simulink model "PolePlacement_Complete"  (R2021a)
settings: Solver=VariableStepAuto  StartTime=0.0  StopTime=10.0  RelTol=1e-3
values from neighbouring files (symbols this model uses):
  k = place(sysestc.A, sysestc.B, new_pole)    [PolePlacement.m]    (also in PolePlacement_Controller_script.m = place(A, B, new_pole); ppObs.m)
  Kr = 1/Kdc(1)    [PolePlacement.m]    (also in PolePlacement_Controller_script.m; ppObs.m)
  L = place(sysestc.A',sysestc.C', 10*new_pole)'    [PolePlacement.m]    (also in PolePlacement_Controller_script.m; ppObs.m)
  sysestc = d2c(sysest)    [PolePlacement.m]    (also in PolePlacement_Controller_script.m; ppObs.m)
undefined symbols (not defined in the file or in its folder): Kp, sigbuilder_block, Ti
libraries: cstblocks x1
settings Model: Creator=jesuc  LastModifiedBy=andre

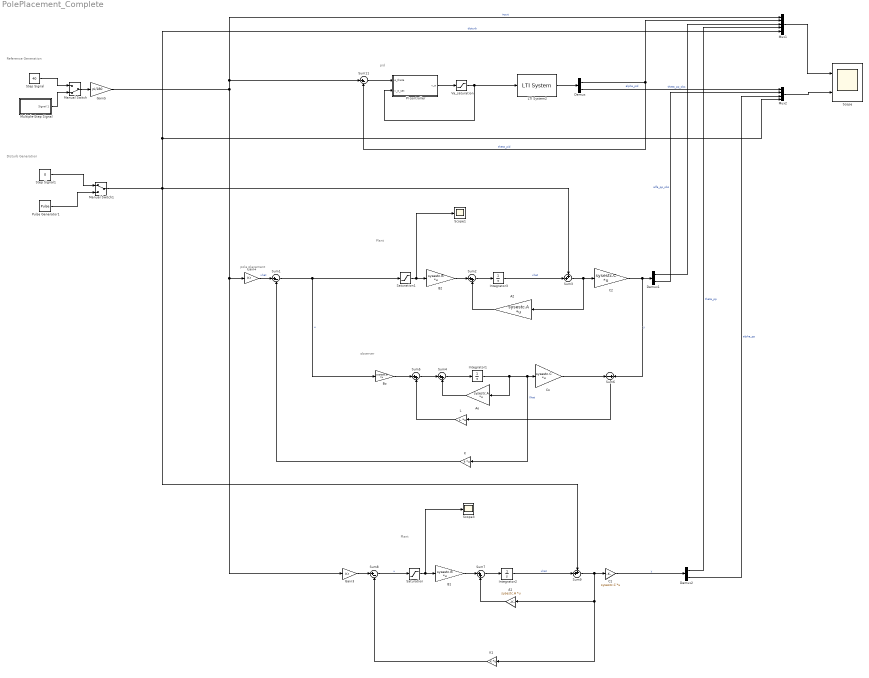
== system PolePlacement_Complete ==
  note: pole placement
  note: observer
  note: Plant
  note: Reference Generation
  note: pid
  note: Plant
  note: Disturb Generation
  A1 : Gain  Gain=sysestc.A  Multiplication=Matrix(K*u)
  A2 : Gain  Gain=sysestc.A  Multiplication=Matrix(K*u)
  Ao : Gain  Gain=sysestc.A  Multiplication=Matrix(K*u)
  B1 : Gain  Gain=sysestc.B  Multiplication=Matrix(K*u)
  B2 : Gain  Gain=sysestc.B  Multiplication=Matrix(K*u)
  Bo : Gain  Gain=sysestc.B  Multiplication=Matrix(K*u)
  C1 : Gain  Gain=sysestc.C  Multiplication=Matrix(K*u)
  C2 : Gain  Gain=sysestc.C  Multiplication=Matrix(K*u)
  Co : Gain  Gain=sysestc.C  Multiplication=Matrix(K*u)
  Demux : Demux  Outputs=2
  Demux1 : Demux  Outputs=2
  Demux2 : Demux  Outputs=2
  Gain3 : Gain  Gain=Kr
  Gain4 : Gain  Gain=Kr
  Gain5 : Gain  Gain=pi/180
  Integrator1 : Integrator
  Integrator2 : Integrator
  Integrator3 : Integrator
  K : Gain  Gain=k  Multiplication=Matrix(K*u)
  K1 : Gain  Gain=k  Multiplication=Matrix(K*u)
  L : Gain  Gain=L  Multiplication=Matrix(K*u)
  LTI System2 : cstblocks/LTI System  sys=sysest  IC=[]
  Manual Switch : ManualSwitch  CurrentSetting=0
  Manual Switch1 : ManualSwitch
  Multiple-Step Signal : Subsystem  Tag=STV Subsys  LoadFcn=sigbuilder_block('load');  StartFcn=sigbuilder_block('start');  StopFcn=sigbuilder_block('stop');  ClipboardFcn=sigbuilder_block('clipboard');  mask(Sigbuilder block){tuvar=[0:10]}
      mask help: Simulink:masks:SigbuilderBlock_MD
      mask init:
      | if ~strcmp(get_param(bdroot(gcbh),'SimulationStatus'),'stopped') tuvar = sigbuilder_block('maskInit'); end
      settings: CopyFcn=sigbuilder_block('copy');  DeleteFcn=sigbuilder_block('delete');  ModelCloseFcn=sigbuilder_block('modelClose');  PreSaveFcn=sigbuilder_block('preSave');  PauseFcn=sigbuilder_block('pause');  ContinueFcn=sigbuilder_block('continue');  NameChangeFcn=sigbuilder_block('namechange');  OpenFcn=sigbuilder_block('open',[437.6 199.2 550.4 400 ]);  CloseFcn=sigbuilder_block('close');
      mask Display: plot(0, 0, 100, 100,[2, 2, 32, 32, 2], [68, 8, 8, 68, 68],[32, 2], [38, 38], [32, 19, 2],[53, 60, 44], [32, 17, 17, 2],[16, 16, 31, 31]);txt = getActiveGroup(gcbh);text(2, 100, txt,'verticalAlignment', 'top');
  Mux1 : Mux  Inputs=5
  Mux2 : Mux
  PI controller : Subsystem
  Pulse Generator1 : DiscretePulseGenerator  PulseType=Time based  Amplitude=.2  Period=1.5  PulseWidth=5
  Saturation : Saturate  UpperLimit=5  LowerLimit=-5
  Saturation1 : Saturate  UpperLimit=5  LowerLimit=-5
  Scope : Scope  NumInputPorts=2
  Scope1 : Scope
  Scope3 : Scope
  Step Signal : Constant  Value=40
  Step Signal1 : Constant  Value=0
  Sum1 : Sum  Inputs=|+-
  Sum11 : Sum  Inputs=|+-
  Sum{2,4..5,7} (4 alike) : Sum  Inputs=|++
  Sum3 : Sum  Inputs=++|
  Sum6 : Sum  Inputs=-+
  Sum8 : Sum  Inputs=|+-
  Sum9 : Sum  Inputs=++|
  Va_saturation : Saturate  UpperLimit=5  LowerLimit=-5
  wires:
  K/1 -> Sum1/2
  Demux1/1 -> Mux1/3  "theta_pp_obs"
  Demux1/2 -> Mux2/2  "alfa_pp_obs"
  Integrator1/1 -> K/1, Co/1, Ao/1  "Xhat"
  L/1 -> Sum5/2
  Sum6/1 -> L/1
  Ao/1 -> Sum4/2
  Co/1 -> Sum6/1
  Sum5/1 -> Sum4/1
  Sum4/1 -> Integrator1/1
  Bo/1 -> Sum5/1
  B1/1 -> Sum7/1
  Sum7/1 -> Integrator2/1
  A1/1 -> Sum7/2
  K1/1 -> Sum8/2
  Sum8/1 -> Saturation/1  "u"
  Gain3/1 -> Sum8/1
  Gain4/1 -> Sum1/1  "xhat"
  Saturation/1 -> B1/1, Scope3/1
  Integrator2/1 -> Sum9/2  "xhat"
  Manual Switch1/1 -> Sum9/1, Mux2/4, Mux1/5, Sum3/1  "disturb"
  Sum9/1 -> K1/1, A1/1, C1/1
  Gain5/1 -> Gain3/1, Gain4/1, Sum11/1, Mux1/1  "input"
  Mux1/1 -> Scope/1
  Demux/1 -> Mux1/2, Sum11/2  "theta_pid"
  Multiple-Step Signal/1(Signal 1) -> Manual Switch/2
  Va_saturation/1 -> LTI System2/1, PI controller/2(v_a_sat)
  Step Signal/1 -> Manual Switch/1
  Manual Switch/1 -> Gain5/1
  PI controller/1(v_a) -> Va_saturation/1
  Sum11/1 -> PI controller/1(e_theta)
  Demux/2 -> Mux2/1  "alpha_pid"
  LTI System2/1 -> Demux/1
  Mux2/1 -> Scope/2
  C1/1 -> Demux2/1  "y"
  Demux2/1 -> Mux1/4  "theta_pp"
  Sum3/1 -> C2/1, A2/1
  Saturation1/1 -> B2/1, Scope1/1
  A2/1 -> Sum2/2
  Integrator3/1 -> Sum3/2  "xhat"
  C2/1 -> Demux1/1, Sum6/2  "y"
  B2/1 -> Sum2/1
  Sum1/1 -> Bo/1, Saturation1/1  "u"
  Sum2/1 -> Integrator3/1
  Demux2/2 -> Mux2/3  "alpha_pp"
  Step Signal1/1 -> Manual Switch1/1
  Pulse Generator1/1 -> Manual Switch1/2

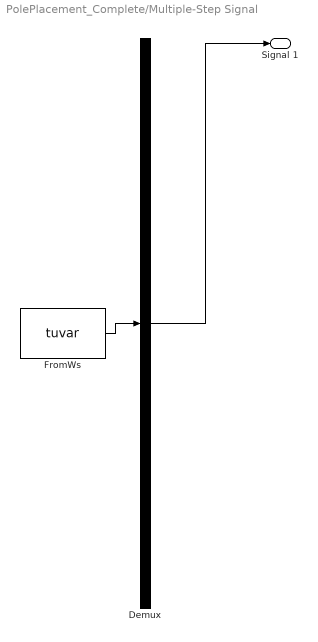
== system PolePlacement_Complete/Multiple-Step Signal ==
  Demux : Demux  Tag=STV Demux  Outputs=1
      settings: DisplayOption=none
  FromWs : FromWorkspace  Tag=STV FromWs  VariableName=tuvar
      SigBuilderData=|
      | common.afterFinalStr = 'Extrapolate'
      | common.sampleTime = 0
      | dataSet.timeRange = [0 10]
      | dataSet.name = 'Group 1'
      | sbobj.Groups.Name = 'Group 1'
      | sbobj.Groups.Signals.Name = 'Signal 1'
      | sbobj.Groups.Signals.XData = [0 1 1 3 3 5 5 7 7 8.5 8.5 10]
      | sbobj.Groups.Signals.YData = [0.005 0.005 40 40 15 15 -30 -30 0 0 23 23]
  Signal 1 : Outport  Tag=STV Outport
  wires:
  Demux/1 -> Signal 1/1
  FromWs/1 -> Demux/1

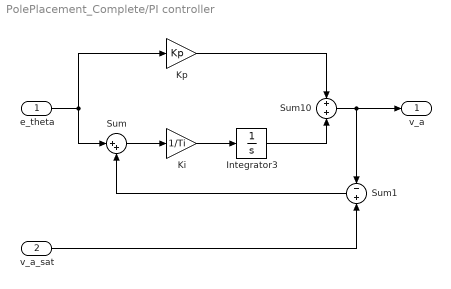
== system PolePlacement_Complete/PI controller ==
  e_theta : Inport
  v_a_sat : Inport  Port=2
  Integrator3 : Integrator
  Ki : Gain  Gain=1/Ti
  Kp : Gain  Gain=Kp
  Sum : Sum  Inputs=|++
  Sum1 : Sum  Inputs=-+
  Sum10 : Sum
  v_a : Outport
  wires:
  e_theta/1 -> Sum/1, Kp/1
  Ki/1 -> Integrator3/1
  Sum10/1 -> v_a/1, Sum1/1
  Integrator3/1 -> Sum10/2
  Kp/1 -> Sum10/1
  Sum/1 -> Ki/1
  v_a_sat/1 -> Sum1/2
  Sum1/1 -> Sum/2
